simulink model "iddempr2"  (Simulink 6.3)
settings: Solver=ode45  StartTime=0.0  StopTime=500  RelTol=1e-3
settings Model: Creator=ljung  LastModifiedBy=rsingh  ExtModeTrigMode=oneshot  ExtModeArmWhenConnect=off  ExtModeAutoUpdateStatusClock=off  StrictBusMsg=None
settings DataIOCC: LimitDataPoints=off
settings OptimizationCC: BooleanDataType=off
settings DebuggingCC: SolverPrmCheckMsg=none  IntegerOverflowMsg=none
settings HardwareCC: TargetUnknown=on

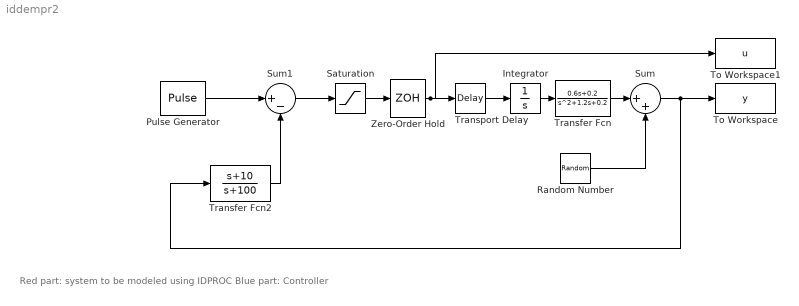
== system iddempr2 ==
  note: Red part: system to be modeled using IDPROC
      | Blue part: Controller
  Integrator : Integrator
  Pulse Generator : DiscretePulseGenerator  Period=200  PulseWidth=50
  Random Number : RandomNumber  Variance=0.1  SampleTime=1
  Saturation : Saturate
  Sum : Sum  Inputs=|++  SaturateOnIntegerOverflow=on  InputSameDT=on
  Sum1 : Sum  Inputs=|+-  SaturateOnIntegerOverflow=on  InputSameDT=on
  To Workspace : ToWorkspace  VariableName=y  SampleTime=1  SaveFormat=Array
  To Workspace1 : ToWorkspace  VariableName=u  SampleTime=1  SaveFormat=Array
  Transfer Fcn : TransferFcn  Numerator=[0.6 0.2]  Denominator="[1 1.2  0.2]"
  Transfer Fcn2 : TransferFcn  Numerator=[1 10]  Denominator=[1 100]
  Transport Delay : TransportDelay  DelayTime=2.2
  Zero-Order Hold : ZeroOrderHold
  wires:
  Transfer Fcn/1 -> Sum/1
  Random Number/1 -> Sum/2
  Sum/1 -> To Workspace/1, Transfer Fcn2/1
  Zero-Order Hold/1 -> To Workspace1/1, Transport Delay/1
  Transport Delay/1 -> Integrator/1
  Integrator/1 -> Transfer Fcn/1
  Sum1/1 -> Saturation/1
  Saturation/1 -> Zero-Order Hold/1
  Transfer Fcn2/1 -> Sum1/2
  Pulse Generator/1 -> Sum1/1
